simulink model "dvbs1_model"  (R2022a)
settings: Solver=VariableStepDiscrete  StartTime=0.0  StopTime=inf  RelTol=1e-3  EnableMultiTasking=on
values from neighbouring files (symbols this model uses):
  M = 4    [errPattern.m]    (also in reprZespolona.m; wsp_szczytu.m)
undefined symbols (not defined in the file or in its folder): EbNodB, rsgenpoly
libraries: simulink x4, commsink2 x3, commblkcod2 x2, commcnvcod2 x2, commcnvintrlv2 x2, commdigbbndpm3 x2, commchan3 x1, impairlib x1, commrandsrc2 x1
settings Model: Creator=Administrator  LastModifiedBy=User
settings SolverCC: AlgebraicLoopSolver=TrustRegion
settings DataIOCC: LimitDataPoints=on  SaveFormat=Array  SignalLoggingSaveFormat=ModelDataLogs  ReturnWorkspaceOutputs=off
settings OptimizationCC: ExpressionDepthLimit=2147483647  InitFltsAndDblsToZero=on  LifeSpan=inf
settings DebuggingCC: UnderspecifiedInitializationDetection=Classic  MergeDetectMultiDrivingBlocksExec=none  SolverPrmCheckMsg=warning  FcnCallInpInsideContextMsg=warning  UnconnectedInputMsg=warning  UnconnectedOutputMsg=warning  UnconnectedLineMsg=warning  StateNameClashWarn=warning  SFUnexpectedBacktrackingDiag=warning  SFNoUnconditionalDefaultTransitionDiag=warning  SFMachineParentedDataDiag=warning  ArithmeticOperatorsInVariantConditions=warning
settings HardwareCC: ProdBitPerPointer=32  ProdBitPerSizeT=32  ProdBitPerPtrDiffT=32  ProdLargestAtomicFloat=None  ProdIntDivRoundTo=Undefined  ProdEndianess=Unspecified  ProdWordSize=32  ProdHWDeviceType=32-bit Generic
settings ModelReferenceCC: PropagateSignalLabelsOutOfModel=off
settings SFSimCC: SimUseLocalCustomCode=off  CustomCodeUndefinedFunction=UseInterfaceOnly
settings RTWCC: RTWUseLocalCustomCode=off
settings CodeAppCC: StateflowObjectComments=on
settings GRTTargetCC: TargetLangStandard=C89/C90 (ANSI)  CombineOutputUpdateFcns=off  GRTInterface=on
settings ConfigComp: CovMetricSettings=dw  CovSaveCumulativeToWorkspaceVar=on  CovSaveSingleToWorkspaceVar=on  CovExternalEMLEnable=off

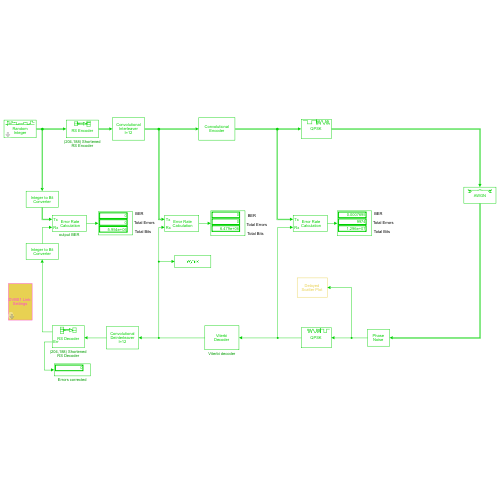
[thumbnail: Simulink's stored preview of the top-level diagram]
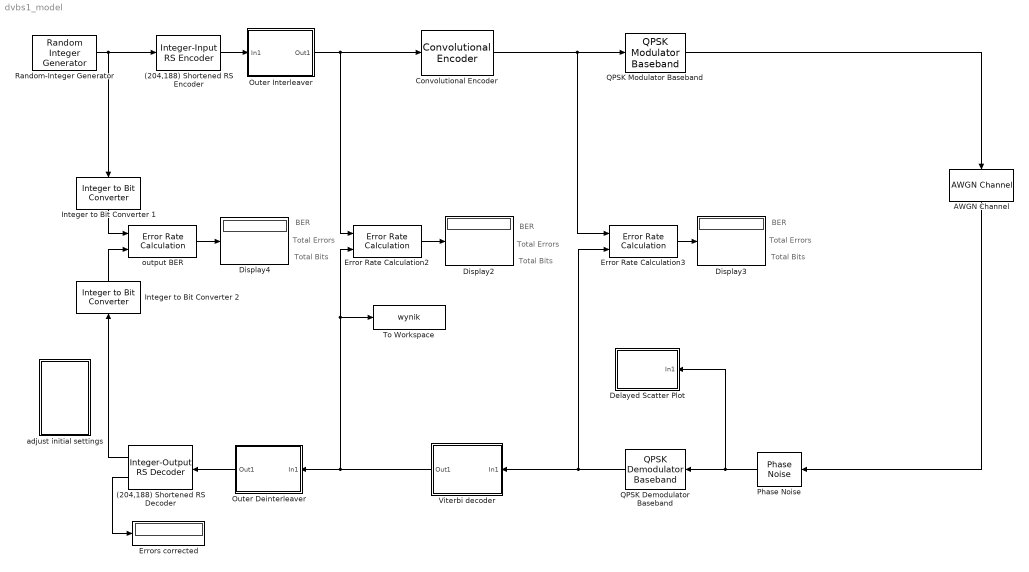
== system dvbs1_model ==
  note: Total Errors
  note: Total Bits
  note: BER
  note: Total Errors
  note: Total Bits
  note: BER
  note: Total Errors
  note: Total Bits
  note: BER
  (204,188) Shortened RS Decoder : commblkcod2/Integer-Output RS Decoder  n=204  k=188  specShortening=off  shortenedK=3  specGenPoly=off  genPoly=rsgenpoly(7,3)  specPrimPoly=off  prPoly=[1 0 1 1]  specPuncture=off  punctVec=[ones(2,1); zeros(2,1)]  specErasurePort=off  showNumErr=on
      settings: SourceProductBaseCode=CM
  (204,188) Shortened RS Encoder : commblkcod2/Integer-Input RS Encoder  n=204  k=188  specShortening=off  shortenedK=3  specGenPoly=off  genPoly=rsgenpoly(7,3)  specPrimPoly=off  prPoly=[1 0 1 1]  specPuncture=off  punctVec=[ones(2,1); zeros(2,1)]
      settings: SourceProductBaseCode=CM
  AWGN Channel : commchan3/AWGN Channel  InputProcessing=Columns as channels (frame based)  seed=54321  noiseMode="Signal to noise ratio  (SNR)"  EbNodB=6  EsNodB=EbNodB+10*log10(log2(M))  SNRdB=10  bitsPerSym=2  Ps=1  Tsym=1  variance=10^(-0.1*15)/(2048*2)
  Convolutional Encoder : commcnvcod2/Convolutional Encoder  trellis=poly2trellis(7, [171 133])  opMode=Continuous  DelayedResetAction=off  hasIniStPort=off  hasFinStPort=off  usePuncVector=off  punctureVector=[1;1;0;1;0;1;0;1;1;0;0;1;1;0]  reset=Unused parameter value
      settings: SourceProductBaseCode=CM
  Delayed Scatter Plot : Subsystem
      mask Display: disp('Delayed\nScatter Plot');
  Display2 : Display
  Display3 : Display
  Display4 : Display
  Error Rate Calculation2 : commsink2/Error Rate Calculation  N=1632  st_delay=0  cp_mode=Entire frame  subframe=[]  PMode=Port  WsName=e1  RsMode2=off  stop=off  numErr=100  maxBits=1e8
  Error Rate Calculation3 : commsink2/Error Rate Calculation  N=0  st_delay=0  cp_mode=Entire frame  subframe=[]  PMode=Port  WsName=BER  RsMode2=off  stop=off  numErr=100  maxBits=1e8
  Errors corrected : Display
  Integer to Bit Converter 1 : simulink/Logic and Bit Operations/Integer to Bit Converter  nbits=8  signedInputValues=Unsigned  bitOrder=MSB first  outDtype=boolean
      settings: SourceProductBaseCode=SL
  Integer to Bit Converter 2 : simulink/Logic and Bit Operations/Integer to Bit Converter  nbits=8  signedInputValues=Unsigned  bitOrder=MSB first  outDtype=boolean
      settings: SourceProductBaseCode=SL
  Outer Deinterleaver : Subsystem  mask(Convolutional Deinterleaver){}
      mask Display: disp('Convolutional\nDeinterleaver\nI=12')
  Outer Interleaver : Subsystem  mask(Convolutional Interleaver){}
      mask Display: disp('Convolutional\nInterleaver\nI=12')
  Phase Noise : impairlib/Phase Noise  Level=-100  FrequencyOffset=100  SampleRate=1024  RandomStream=mt19937ar with seed  Seed=2137  SimulateUsing=Interpreted execution
      settings: SourceProductBaseCode=CM,AM,SX
  QPSK Demodulator Baseband : commdigbbndpm3/QPSK Demodulator Baseband  OutType=Bit  DecType=Hard decision  VarSource=Dialog  Variance=1  Dec=Gray  Ph=pi/4  outDtype1=boolean  outDtype2=Inherit via internal rule  derotateFactorWordLen=16  derotateFactorDataTypeStr=Inherit: Same word length as input  derotateFactorLastDataTypeStr=Inherit: Same word length as input
  QPSK Modulator Baseband : commdigbbndpm3/QPSK Modulator Baseband  InType=Bit  Enc=Gray  Ph=pi/4  outDtype=double  outWordLen=16  outUDDataType=sfix(16)  outFracLenMode=Best precision  outFracLen=15  outDataTypeStr=double  outLastDataTypeStr=double
  Random-Integer Generator : commrandsrc2/Random Integer Generator  mul=256  seed=1234573  Ts=8*(204/188)  frameBased=on  sampPerFrame=188  orient=off  outDataType=uint8
      settings: SourceProductBaseCode=CM
  To Workspace : ToWorkspace  VariableName=wynik  SampleTime=-1
      settings: Save2DSignal=2-D array (concatenate along first dimension)
  Viterbi decoder : Subsystem
      mask Display: disp('Viterbi\nDecoder')
  adjust initial settings : Subsystem  mask(RF Link Demo:Initial Settings){selNoPh=Negligible (-100 dBc/Hz @ 100 Hz), CodeRate=1/2, test=10}
      mask prompts: selNoPh "Phase noise:"; CodeRate "FEC code rate:"; test "EbNo:"
      mask help: Select the scenarios from the mask to change the link parameters. Each of the mask parameters sets the parameters in the corresponding RF impairment block(s).
      mask init:
      | EbNo=test-1;
      | codeRate=0.5;
      | set_param('dvbs1_model/AWGN Channel','SNRdB',sprintf('%g',EbNo+10*log10(2.0*codeRate)))
      | 
      | switch selNoPh
      |     case 1,
      |     set_param('dvbs1_model/Phase Noise','Level','-100')
      |     case 2,
      |     set_param('dvbs1_model/Phase Noise','Level','-55')
      |     case 3,    
      |     set_param('dvbs1_model/Phase Noise','Level','-48')
      | end
      | 
      |    switch CodeRate
      |         case 1, %1/2
      |         codeRate=0.5;
      |         set_param('dvbs1_model/Convolutional Encoder','usePuncVector','off')
      |         set_param('dvbs1_model/Viterbi decoder/Viterbi Decoder','isPunctured','off')
      |         set_param('dvbs1_model/Random-Integer Generator','sampPerFrame','188')
      | 
      |         case 2, %2/3
      |         codeRate=0.66;
      |         set_param('dvbs1_model/Convolutional Encoder','usePuncVector','on')
      |         set_param('dvbs1_model/Convolutional Encoder','punctureVector','[1; 1; 0; 1]')
      |         set_param('dvbs1_model/Viterbi decoder/Viterbi Decoder','isPunctured','on')
      |         set_param('dvbs1_model/Viterbi decoder/Viterbi Decoder','punctureVector','[1; 1; 0; 1]')
      |         set_param('dvbs1_model/AWGN Channel','SNRdB',sprintf('EbNo + %g',10*log10(2.0*codeRate)))        
      |         set_param('dvbs1_model/Random-Integer Generator','sampPerFrame','188')
      |         case 3, %3/4
      |         codeRate=0.75;
      |         set_param('dvbs1_model/Convolutional Encoder','usePuncVector','on')
      |         set_param('dvbs1_model/Convolutional Encoder','punctureVector','[1; 1; 0; 1; 1; 0]')
      |         set_param('dvbs1_model/Viterbi decoder/Viterbi Decoder','isPunctured','on')
      |         set_param('dvbs1_model/Viterbi decoder/Viterbi Decoder','punctureVector','[1; 1; 0; 1; 1; 0]')
      |         set_param('dvbs1_model/Random-Integer Generator','sampPerFrame','188')
      |         case 4, %5/6
      |         codeRate=0.83;            
      |         set_param('dvbs1_model/Convolutional Encoder','usePuncVector','on')
      |         set_param('dvbs1_model/Convolutional Encoder','punctureVector','[1; 1; 0; 1; 1; 0; 0; 1;1;0]')
      |         set_param('dvbs1_model/Viterbi decoder/Viterbi Decoder','isPunctured','on')
      |         set_param('dvbs1_model/Viterbi decoder/Viterbi Decoder','punctureVector','[1; 1; 0; 1; 1; 0; 0; 1;1;0]')
      |         set_param('dvbs1_model/Random-Integer Generator','sampPerFrame','188*5')
      |         case 5, %7/8
      |         codeRate=0.875;            
      |         set_param('dvbs1_model/Convolutional Encoder','usePuncVector','on')
      |         set_param('dvbs1_model/Convolutional Encoder','punctureVector','[1;1;0;1;0;1;0;1;1;0;0;1;1;0]')
      |         set_param('dvbs1_model/Viterbi decoder/Viterbi Decoder','isPunctured','on')
      |         set_param('dvbs1_model/Viterbi decoder/Viterbi Decoder','punctureVector','[1;1;0;1;0;1;0;1;1;0;0;1;1;0]')
      |         set_param('dvbs1_model/Random-Integer Generator','sampPerFrame','188*7')
      |    end
      | set_param('dvbs1_model/AWGN Channel','SNRdB',sprintf('%g',EbNo + 10*log10(2.0*codeRate)))
      mask TypeOptions selNoPh: Negligible (-100 dBc/Hz @ 100 Hz) | Low  (-55 dBc/Hz @ 100 Hz) | High  (-48 dBc/Hz @ 100 Hz)
      mask TypeOptions CodeRate: 1/2 | 2/3 | 3/4 | 5/6 | 7/8
      mask TypeOptions test: 0 | 1 | 2 | 3 | 4 | 5 | 6 | 7 | 8 | 9 | 10
      mask Display: disp('DVBS1 Link:\nSettings');
  output BER : commsink2/Error Rate Calculation  N=188*8*12  st_delay=0  cp_mode=Entire frame  subframe=[]  PMode=Port  WsName=e1  RsMode2=off  stop=off  numErr=100  maxBits=1e6
  wires:
  (204,188) Shortened RS Encoder/1 -> Outer Interleaver/1(In1)
  Outer Interleaver/1(Out1) -> Convolutional Encoder/1, Error Rate Calculation2/1
  QPSK Modulator Baseband/1 -> AWGN Channel/1
  QPSK Demodulator Baseband/1 -> Viterbi decoder/1(In1), Error Rate Calculation3/2
  Outer Deinterleaver/1(Out1) -> (204,188) Shortened RS Decoder/1
  Error Rate Calculation2/1 -> Display2/1
  (204,188) Shortened RS Decoder/1 -> Integer to Bit Converter 2/1
  Convolutional Encoder/1 -> QPSK Modulator Baseband/1, Error Rate Calculation3/1
  Random-Integer Generator/1 -> (204,188) Shortened RS Encoder/1, Integer to Bit Converter 1/1
  output BER/1 -> Display4/1
  Integer to Bit Converter 1/1 -> output BER/1
  Integer to Bit Converter 2/1 -> output BER/2
  Phase Noise/1 -> QPSK Demodulator Baseband/1, Delayed Scatter Plot/1(In1)
  Error Rate Calculation3/1 -> Display3/1
  (204,188) Shortened RS Decoder/2 -> Errors corrected/1
  Viterbi decoder/1(Out1) -> Outer Deinterleaver/1(In1), To Workspace/1, Error Rate Calculation2/2
  AWGN Channel/1 -> Phase Noise/1

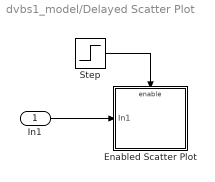
== system dvbs1_model/Delayed Scatter Plot ==
  In1 : Inport
  Enabled Scatter Plot : Subsystem  TreatAsAtomicUnit=on
  Step : Step  Time=.001  SampleTime=1
  wires:
  Step/1 -> Enabled Scatter Plot/Enable
  In1/1 -> Enabled Scatter Plot/1(In1)

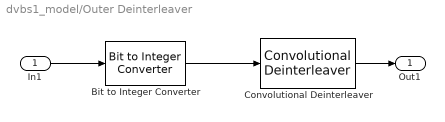
== system dvbs1_model/Outer Deinterleaver ==
  In1 : Inport
  Bit to Integer Converter : simulink/Logic and Bit Operations/Bit to Integer Converter  nbits=8  bitOrder=MSB first  signedOutputValues=Unsigned  outDtype=uint8  outDtypeSigned=Inherit via internal rule
      settings: SourceProductBaseCode=SL
  Convolutional Deinterleaver : commcnvintrlv2/Convolutional Deinterleaver  N=12  B=17  ic=0
      settings: SourceProductBaseCode=CM
  Out1 : Outport
  wires:
  In1/1 -> Bit to Integer Converter/1
  Convolutional Deinterleaver/1 -> Out1/1
  Bit to Integer Converter/1 -> Convolutional Deinterleaver/1

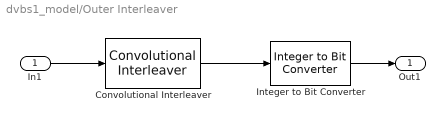
== system dvbs1_model/Outer Interleaver ==
  In1 : Inport
  Convolutional Interleaver : commcnvintrlv2/Convolutional Interleaver  N=12  B=17  ic=0
      settings: SourceProductBaseCode=CM
  Integer to Bit Converter : simulink/Logic and Bit Operations/Integer to Bit Converter  nbits=8  signedInputValues=Unsigned  bitOrder=MSB first  outDtype=boolean
      settings: SourceProductBaseCode=SL
  Out1 : Outport
  wires:
  Integer to Bit Converter/1 -> Out1/1
  Convolutional Interleaver/1 -> Integer to Bit Converter/1
  In1/1 -> Convolutional Interleaver/1

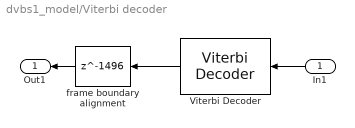
== system dvbs1_model/Viterbi decoder ==
  In1 : Inport
  " frame boundary alignment" : Delay  DelayLength=1496  InitialCondition=0  InputProcessing=Columns as channels (frame based)
  Viterbi Decoder : commcnvcod2/Viterbi Decoder  trellis=poly2trellis(7, [171 133])  isPunctured=off  punctureVector=[1;1;0;1;0;1;0;1;1;0;0;1;1;0]  erasures=off  dectype=Hard decision  nsdecb=4  runSigValErrCheck=off  tbdepth=136  opmode=Continuous  reset=off  delayedResetAction=off  smWordLength=16  outDataType=boolean
      settings: SourceProductBaseCode=CM
  Out1 : Outport
  wires:
  Viterbi Decoder/1 -> " frame boundary alignment"/1
  In1/1 -> Viterbi Decoder/1
  " frame boundary alignment"/1 -> Out1/1

== system dvbs1_model/adjust initial settings ==

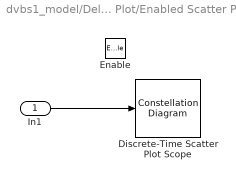
== system dvbs1_model/Delayed Scatter Plot/Enabled Scatter Plot ==
  In1 : Inport
  Enable : EnablePort
  Discrete-Time Scatter Plot Scope : ConstellationDiagram  Tag=ScatterPlot  WindowPosition=[1097.000000,525.000000,410.000000,300.000000,]  ScopeFrameLocation=window  DefaultConfigurationName=comm.scopes.ConstellationDiagramBlockCfg
  wires:
  In1/1 -> Discrete-Time Scatter Plot Scope/1
